simulink model "tadpole_dynamic_open_loop1"  (R2019b)
settings: Solver=ode4  StartTime=0.0  StopTime=sim_time  FixedStep=0.001  RelTol=1e-2
values from neighbouring files (symbols this model uses):
  C_alpha = 1000*ones(runcycle,1)    [rand_par.m]    (also in whole_par.m = 1000; whole_par_bias.m = 1000)
  C_beta = 50*ones(runcycle,1)    [rand_par.m]    (also in whole_par.m = 50; whole_par_bias.m = 50)
  Cd = 0.25*ones(runcycle,1)    [rand_par.m]    (also in whole_par.m = 0.25; whole_par_bias.m = 0.25)
  delta_fL = -1*ones(runcycle,1)    [rand_par.m]    (also in whole_par.m = -1; whole_par_bias.m = -1)
  delta_fR = 3.5*ones(runcycle,1)    [rand_par.m]    (also in whole_par.m = 3.5; whole_par_bias.m = 3.5)
  FA = 1*ones(runcycle,1)    [rand_par.m]    (also in whole_par.m = 1; whole_par_bias.m = 1)
  h = [ h(1:j-1) ; h(j+1:m)]    [UMDIRECT.m]    (also in whole_par.m = 0.4896; whole_par_bias.m = 0.4896)
  I_f_wheel = 0.3    [whole_par.m]    (also in whole_par_bias.m)
  I_r_wheel = 0.5    [whole_par.m]    (also in whole_par_bias.m)
  I_x = 12.1*ones(runcycle,1)    [rand_par.m]    (also in whole_par.m = 12.1; whole_par_bias.m = 12.1)
  I_y = 36.7*ones(runcycle,1)    [rand_par.m]    (also in whole_par.m = 36.7; whole_par_bias.m = 36.7)
  I_z = 50*DOE(:,2)    [rand_par.m]    (also in whole_par.m = 50; whole_par_bias.m = 60)
  k_z = 30000*ones(runcycle,1)    [rand_par.m]    (also in whole_par.m = 30000; whole_par_bias.m = 30000)
  l_1 = 0.724    [whole_par.m]    (also in whole_par_bias.m)
  l_2 = 0.719    [whole_par.m]    (also in whole_par_bias.m)
  m = m - 1    [UMDIRECT.m]    (also in rand_par.m = 48.3*DOE(:,1); whole_par.m = 48.3; whole_par_bias.m = 60)
  mu_dp = 0.8*ones(runcycle,1)    [rand_par.m]    (also in whole_par.m = 0.8; whole_par_bias.m = 0.8)
  mu_lp = 0.8*ones(runcycle,1)    [rand_par.m]    (also in whole_par.m = 0.8; whole_par_bias.m = 0.8)
  mu_rolling_1 = 0.009*ones(runcycle,1)    [rand_par.m]    (also in whole_par.m = 0.009; whole_par_bias.m = 0.009)
  mu_rolling_2 = 0.0005*ones(runcycle,1)    [rand_par.m]    (also in whole_par.m = 0.0005; whole_par_bias.m = 0.0005)
  R_0 = 0.335*ones(runcycle,1)    [rand_par.m]    (also in whole_par.m = 0.335; whole_par_bias.m = 0.335)
  rho = 1.225*ones(runcycle,1)    [rand_par.m]    (also in whole_par.m = 1.225; whole_par_bias.m = 1.225)
  SAP = 0.01*ones(runcycle,1)    [rand_par.m]    (also in whole_par.m = 0.01; whole_par_bias.m = 0.01)
  V_wind = 0*ones(runcycle,1)    [rand_par.m]    (also in whole_par.m = 0; whole_par_bias.m = 0)
libraries: simulink_extras x10, simulink x4
(part 1 of 4)
settings Model: Creator=yipin  LastModifiedBy=Chenyp
settings SolverCC: ZeroCrossAlgorithm=Adaptive  AlgebraicLoopSolver=LineSearch
settings DataIOCC: ReturnWorkspaceOutputs=off
settings DebuggingCC: MaxConsecutiveZCsMsg=warning  ArithmeticOperatorsInVariantConditions=warning
settings SFSimCC: CustomCodeUndefinedFunction=UseInterfaceOnly

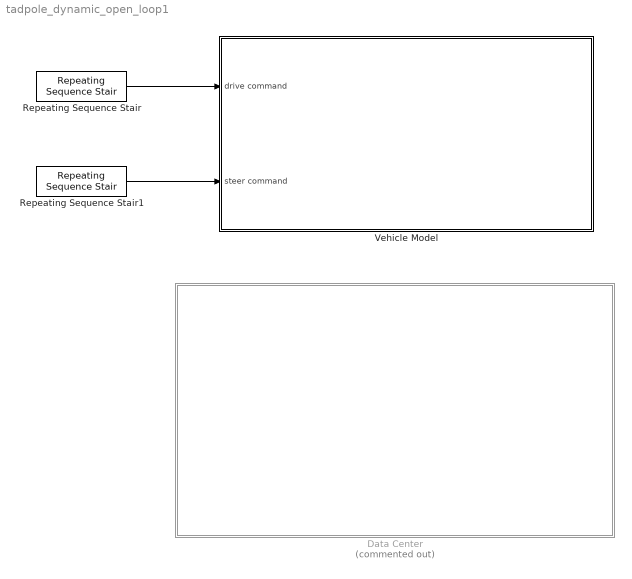
== system tadpole_dynamic_open_loop1 ==
  Data Center : Subsystem  Commented=on
  Repeating Sequence Stair : simulink/Sources/Repeating Sequence Stair  OutValues=drive_command  tsamp=-1  OutMin=[]  OutMax=[]  OutDataTypeStr=double  OutputDataTypeScalingMode=double  OutDataType=fixdt(0,8)  ConRadixGroup=Best Precision: Vector-wise  OutScaling=2^-12
  Repeating Sequence Stair1 : simulink/Sources/Repeating Sequence Stair  OutValues=steer_command  tsamp=-1  OutMin=[]  OutMax=[]  OutDataTypeStr=double  OutputDataTypeScalingMode=double  OutDataType=fixdt(0,8)  ConRadixGroup=Best Precision: Vector-wise  OutScaling=2^-12
  Vehicle Model : Subsystem
      mask Display: image('C:\Users\yipin\Desktop\擷取.PNG');
  wires:
  Repeating Sequence Stair/1 -> Vehicle Model/1("drive command ")
  Repeating Sequence Stair1/1 -> Vehicle Model/2(steer command)

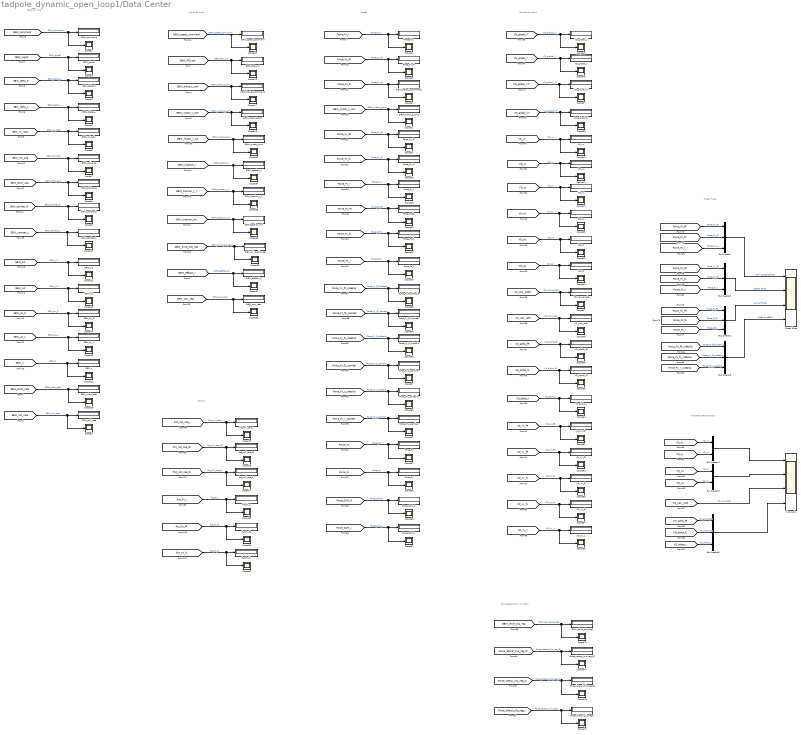
== system tadpole_dynamic_open_loop1/Data Center ==
  note: Steer By Wire
  note: Drive By Wire
  note: Vehicle Dynamic
  note: Forces
  note: Friction
  note: Wheel Force
  note: Kinematic Performance
  note: Slip Recgonition (-1 if slip)
  Bus Creator{,1..3,6} (5 alike) : BusCreator  Inputs=3
  Bus Creator4 : BusCreator  Inputs=2
  Bus Creator5 : BusCreator  Inputs=2
  DBW_PID_out : Display
  DBW_brake_t_command : Display
  DBW_brake_t_command1 : Display
  DBW_drive_slip_reg : Display
  DBW_drive_slip_reg1 : Display
  DBW_effRadi_R : Display
  DBW_motor_t_com : Display
  DBW_motor_t_com1 : Display
  DBW_motor_t_out : Display
  DBW_rpm_rear : Display
  DBW_speed_command : Display
  DBW_traction_out : Display
  DBW_traction_r : Display
  DBW_traction_r_T : Display
  Force_Fx : Display
  Force_Fx_fR : Display
  Force_Fx_r : Display
  Force_Fy : Display
  Force_Fy_fL : Display
  Force_Fy_fL_camber : Display
  Force_Fy_fL_sideslip : Display
  Force_Fy_fR : Display
  Force_Fy_fR_camber : Display
  Force_Fy_fR_sideslip : Display
  Force_Fy_r : Display
  Force_Fy_r_camber : Display
  Force_Fy_r_sideslip : Display
  Force_Fz_fL : Display
  Force_Fz_fR : Display
  Force_Fz_r : Display
  Force_SAM_L : Display
  Force_SAM_R : Display
  Force_lateral_slip_reg_fL : Display
  Force_lateral_slip_reg_fR : Display
  Force_lateral_slip_reg_r : Display
  SBW_an_L : Display
  SBW_an_R : Display
  SBW_camber_L : Display
  SBW_camber_R : Display
  SBW_command : Display
  SBW_delta_L : Display
  SBW_delta_R : Display
  SBW_h : Display
  SBW_pitch_ang : Display
  SBW_pitch_rate : Display
  SBW_roll_ang : Display
  SBW_roll_rate : Display
  SBW_signal : Display
  SBW_w1 : Display
  SBW_w2 : Display
  SBW_wl_ratio : Display
  Scope{1..64,66..68,73..82} (77 alike) : Scope
  VD_Ax : Display
  VD_Ay : Display
  VD_Az : Display
  VD_Vx_fL : Display
  VD_Vx_fR : Display
  VD_Vy_fL : Display
  VD_Vy_fR : Display
  VD_Vy_r : Display
  VD_alpha_fL : Display
  VD_alpha_fR : Display
  VD_alpha_r : Display
  VD_global_VX : Display
  VD_global_VY : Display
  VD_global_X : Display
  VD_global_Y : Display
  VD_vx : Display
  VD_vy : Display
  VD_vz : Display
  VD_yaw_angle : Display
  VD_yaw_rate : Display
  frct_Fx_fL : Display
  frct_Fx_fR : Display
  frct_Fx_r : Display
  frct_roll_coe_fL : Display
  frct_roll_coe_fR : Display
  frct_roll_coe_r : Display
  "kinematic " : Scope  NumInputPorts=4
  wheel force : Scope  NumInputPorts=4
  wires:
  [SBW_wl_ratio] -> Scope6/1, SBW_wl_ratio/1  "SBW_wl_ratio"
  [SBW_w2] -> Scope13/1, SBW_w2/1  "SBW_w2"
  [SBW_delta_L] -> Scope5/1, SBW_delta_L/1  "SBW_delta_L"
  [SBW_camber_R] -> Scope9/1, SBW_camber_R/1  "SBW_camber_R"
  [SBW_w1] -> Scope12/1, SBW_w1/1  "SBW_w1"
  [SBW_an_R] -> Scope14/1, SBW_an_R/1  "SBW_an_R"
  [SBW_signal] -> Scope3/1, SBW_signal/1  "SBW_signal"
  [SBW_pitch_ang] -> Scope8/1, SBW_pitch_ang/1  "SBW_pitch_ang"
  [SBW_an_L] -> Scope15/1, SBW_an_L/1  "SBW_an_L"
  [SBW_camber_L] -> Scope10/1, SBW_camber_L/1  "SBW_camber_L"
  [SBW_command] -> Scope1/1, SBW_command/1  "SBW_command"
  [SBW_delta_R] -> Scope4/1, SBW_delta_R/1  "SBW_dalta_R"
  [SBW_h] -> Scope11/1, SBW_h/1  "SBW_h"
  [SBW_roll_ang] -> Scope7/1, SBW_roll_ang/1  "SBW_roll_ang"
  [SBW_pitch_rate] -> Scope16/1, SBW_pitch_rate/1  "SBW_pitch_rate"
  [SBW_roll_rate] -> Scope2/1, SBW_roll_rate/1  "SBW_roll_rate"
  [DBW_PID_out] -> Scope19/1, DBW_PID_out/1  "DBW_PID_out"
  [DBW_motor_t_com] -> Scope18/1, DBW_motor_t_com/1  "DBW_motor_t_com"
  [DBW_brake_t_com] -> Scope17/1, DBW_brake_t_command/1  "DBW_brake_t_com"
  [DBW_speed_command] -> Scope20/1, DBW_speed_command/1  "DBW_speed_command"
  [Force_Fx_r] -> Scope24/1, Force_Fx_r/1  "Force_Fx_r"
  [DBW_motor_t_com] -> Scope22/1, DBW_motor_t_com1/1  "DBW_motor_t_com"
  [Force_Fx_fL] -> Scope21/1, DBW_brake_t_command1/1  "Force_Fx_fL"
  [Force_Fx_fR] -> Scope23/1, Force_Fx_fR/1  "Force_Fx_fR"
  [Force_Fy_fR] -> Scope27/1, Force_Fy_fR/1  "Force_Fy_fR"
  [Force_Fy_r] -> Scope26/1, Force_Fy_r/1  "Force_Fy_r"
  [Force_Fy_fL] -> Scope25/1, Force_Fy_fL/1  "Force_Fy_fL"
  [Force_Fz_r] -> Scope29/1, Force_Fz_r/1  "Force_Fz_r"
  [Force_Fz_fR] -> Scope30/1, Force_Fz_fR/1  "Force_Fz_fR"
  [Force_Fz_fL] -> Scope28/1, Force_Fz_fL/1  "Force_Fz_fL"
  [DBW_effRadi_r] -> Scope31/1, DBW_effRadi_R/1  "DBW_effRadi_R"
  [DPW_rpm_rear] -> Scope32/1, DBW_rpm_rear/1  "DBW_rpm_rear"
  [DBW_motor_t_out] -> Scope33/1, DBW_motor_t_out/1  "DBW_motor_t_out"
  [DBW_traction_r] -> Scope34/1, DBW_traction_r/1  "DBW_traction_r"
  [DBW_traction_r_T] -> Scope35/1, DBW_traction_r_T/1  "DBW_traction_r_T"
  [DBW_drive_slip_reg] -> Scope36/1, DBW_drive_slip_reg/1  "DBW_drive_slip_reg"
  [VD_Ay] -> Scope43/1, VD_Ay/1  "VD_Ay"
  [VD_Ax] -> Scope38/1, VD_Ax/1  "VD_Ax"
  [VD_global_VX] -> Scope37/1, VD_global_VX/1  "VD_global_VX"
  [VD_vz] -> Scope42/1, VD_vz/1  "VD_vz"
  [VD_global_VY] -> Scope39/1, VD_global_VY/1  "VD_global_VY"
  [VD_vy] -> Scope41/1, VD_vy/1  "VD_vy"
  [VD_vx] -> Scope40/1, VD_vx/1  "VD_vx"
  [VD_global_X] -> Scope45/1, VD_global_X/1  "VD_global_X"
  [VD_global_Y] -> Scope46/1, VD_global_Y/1  "VD_global_Y"
  [VD_Az] -> Scope44/1, VD_Az/1  "VD_Az"
  [VD_yaw_rate] -> Scope48/1, VD_yaw_rate/1  "VD_yaw_rate"
  [VD_yaw_angle] -> Scope47/1, VD_yaw_angle/1  "VD_yaw_angle"
  [VD_alpha_fR] -> Scope49/1, VD_alpha_fR/1  "VD_alpha_fR"
  [VD_alpha_fL] -> Scope50/1, VD_alpha_fL/1  "VD_alpha_fL"
  [VD_Vx_fL] -> Scope53/1, VD_Vx_fL/1  "VD_Vx_fL"
  [VD_Vy_fL] -> Scope54/1, VD_Vy_fL/1  "VD_Vy_fL"
  [VD_Vx_fR] -> Scope51/1, VD_Vx_fR/1  "VD_Vx_fR"
  [VD_Vy_fR] -> Scope52/1, VD_Vy_fR/1  "VD_Vy_fR"
  [Force_Fy_fR_sideslip] -> Scope55/1, Force_Fy_fR_sideslip/1  "Force_Fy_fR_sideslip"
  [Force_Fy_fR_camber] -> Scope58/1, Force_Fy_fR_camber/1  "Force_Fy_fR_camber"
  [Force_Fy_fL_sideslip] -> Scope56/1, Force_Fy_fL_sideslip/1  "Force_Fy_fL_sideslip"
  [Force_Fy_fL_camber] -> Scope57/1, Force_Fy_fL_camber/1  "Force_Fy_fL_camber"
  [VD_Vy_r] -> Scope59/1, VD_Vy_r/1  "VD_Vy_r"
  [Force_Fy_r_camber] -> Scope61/1, Force_Fy_r_camber/1  "Force_Fy_r_camber"
  [Force_Fy_r_sideslip] -> Scope60/1, Force_Fy_r_sideslip/1  "Force_Fy_r_sideslip"
  [Force_Fx] -> Scope62/1, Force_Fx/1  "Force_Fx"
  [Force_Fy] -> Scope63/1, Force_Fy/1  "Force_Fy"
  [Force_SAM_L] -> Scope67/1, Force_SAM_L/1  "Force_SAM_L"
  [Force_SAM_R] -> Scope66/1, Force_SAM_R/1  "Force_SAM_R"
  [DBW_traction_out] -> Scope68/1, DBW_traction_out/1  "DBW_traction_out"
  [Force_Fx_r_r] -> Bus Creator/3  "Force_Fx_r_r"
  [Force_Fx_fL] -> Bus Creator/2  "Force_Fx_fL"
  [Force_Fx_fR] -> Bus Creator/1  "Force_Fx_fR"
  [Force_Fy_fR] -> Bus Creator1/1  "Force_Fy_fR"
  [Force_Fy_fL] -> Bus Creator1/2  "Force_Fy_fL"
  [Force_Fz_fR] -> Bus Creator2/1  "Force_Fz_fR"
  [Force_Fz_fL] -> Bus Creator2/2  "Force_Fz_fL"
  [Force_Fz_r] -> Bus Creator2/3  "Force_Fz_r"
  [Force_Fy_fL_sideslip] -> Bus Creator3/2  "Force_Fy_fL_sideslip"
  [Force_Fy_fR_sideslip] -> Bus Creator3/1  "Force_Fy_fR_sideslip"
  [Force_Fy_r_sideslip] -> Bus Creator3/3  "Force_Fy_r_sideslip"
  Bus Creator/1 -> wheel force/1  "Rolling Resistance"
  Bus Creator1/1 -> wheel force/2  "Lateral Force"
  Bus Creator2/1 -> wheel force/3  "Normal Force"
  Bus Creator3/1 -> wheel force/4  "Sideslip effect"
  [Force_Fy_r] -> Bus Creator1/3  "Force_Fy_r"
  [VD_vy] -> Bus Creator4/2  "VD_vy"
  [VD_vx] -> Bus Creator4/1  "VD_vx"
  [VD_Ax] -> Bus Creator5/1  "VD_Ax"
  [VD_Ay] -> Bus Creator5/2  "VD_Ay"
  [VD_alpha_fR] -> Bus Creator6/1  "VD_alpha_fR"
  [VD_alpha_fL] -> Bus Creator6/2  "VD_alpha_fL"
  Bus Creator4/1 -> "kinematic "/1
  Bus Creator5/1 -> "kinematic "/2
  [VD_yaw_rate] -> "kinematic "/3  "VD_yaw_rate"
  Bus Creator6/1 -> "kinematic "/4
  [VD_alpha_r] -> Scope64/1, VD_alpha_r/1  "VD_alpha_r"
  [VD_alpha_r] -> Bus Creator6/3  "VD_alpha_r"
  [DBW_drive_slip_reg] -> Scope73/1, DBW_drive_slip_reg1/1  "DBW_drive_slip_reg"
  [Force_lateral_slip_reg_fR] -> Scope74/1, Force_lateral_slip_reg_fR/1  "Force_lateral_slip_reg_fR"
  [Force_lateral_slip_reg_fL] -> Scope75/1, Force_lateral_slip_reg_fL/1  "Force_lateral_slip_reg_fL"
  [Force_lateral_slip_reg_r] -> Scope76/1, Force_lateral_slip_reg_r/1  "Force_lateral_slip_reg_r"
  [frct_roll_coe_fL] -> Scope77/1, frct_roll_coe_fL/1  "frct_roll_coe_fL"
  [frct_roll_coe_fR] -> Scope78/1, frct_roll_coe_fR/1  "frct_roll_coe_fR"
  [frct_roll_coe_r] -> Scope79/1, frct_roll_coe_r/1  "frct_roll_coe_r"
  [frct_Fx_r] -> Scope80/1, frct_Fx_r/1  "frct_Fx_r"
  [frct_Fx_fR] -> Scope81/1, frct_Fx_fR/1  "frct_Fx_fR"
  [frct_Fx_fL] -> Scope82/1, frct_Fx_fL/1  "frct_Fx_fL"

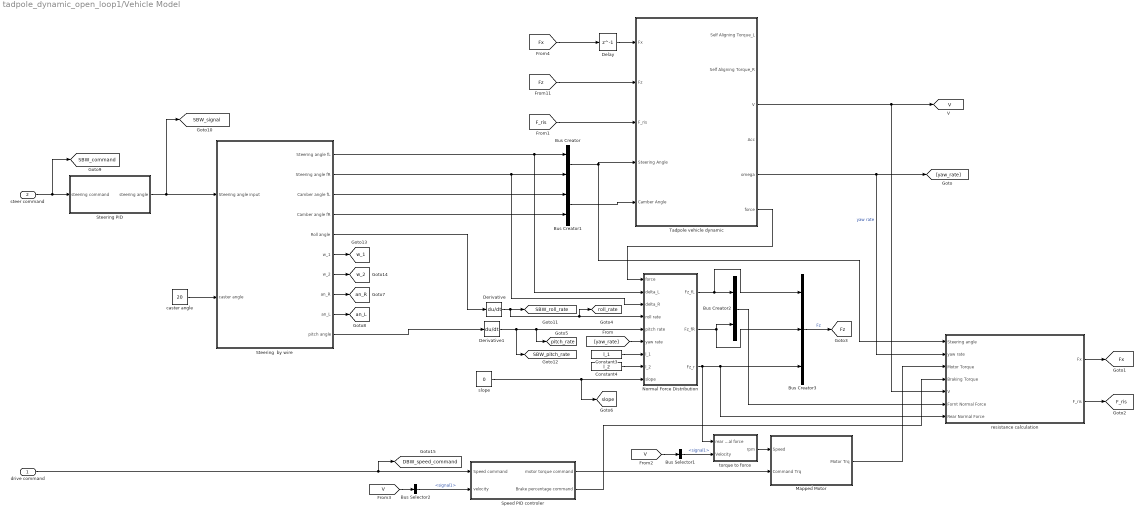
== system tadpole_dynamic_open_loop1/Vehicle Model ==
  "drive command " : Inport
  steer command : Inport  Port=2
  Bus Creator : BusCreator  Inputs=2
  Bus Creator1 : BusCreator  Inputs=2
  Bus Creator2 : BusCreator  Inputs=2
  Bus Creator3 : BusCreator  Inputs=3
  Bus Selector1 : BusSelector  OutputSignals=signal1
  Bus Selector2 : BusSelector  OutputSignals=signal1
  Constant3 : Constant  Value=l_1
  Constant4 : Constant  Value=l_2
  Delay : Delay  DelayLength=1  SampleTime=0.01
  Derivative : Derivative
  Derivative1 : Derivative
  Mapped Motor : Subsystem
  Normal Force Distribution : Subsystem
  "Speed PID controler " : Subsystem
  Steering  by wire : Subsystem  SystemSampleTime=469.048
  Steering PID : Subsystem
  Tadpole vehicle dynamic : Subsystem
  caster angle : Constant  Value=20
  resistance calculation : Subsystem
  slope : Constant  Value=0
  torque to force : Subsystem
  tag scope: DBW_speed_command=global, F_ris=global, Fx=global, Fz=global, SBW_command=global, SBW_pitch_rate=global, SBW_roll_rate=global, SBW_signal=global, V=global, an_L=global, an_R=global, pitch_rate=global, roll_rate=global, slope=global, w_1=global, w_2=global
  wires:
  Steering PID/1("steering angle ") -> [SBW_signal], Steering  by wire/1(Steering angle input)
  Bus Creator/1 -> Tadpole vehicle dynamic/4(Steering Angle), resistance calculation/1(Steering angle)
  Steering  by wire/2(Steering angle fR) -> Normal Force Distribution/3(delta_R), Bus Creator/2
  Steering  by wire/1(Steering angle fL) -> Normal Force Distribution/2(delta_L), Bus Creator/1
  steer command/1 -> [SBW_command], Steering PID/1(steering command)
  caster angle/1 -> Steering  by wire/2(caster angle)
  Steering  by wire/3(Camber angle fL) -> Bus Creator1/1
  Steering  by wire/4(Camber angle fR) -> Bus Creator1/2
  Bus Creator1/1 -> Tadpole vehicle dynamic/5(Camber Angle)
  Tadpole vehicle dynamic/5(omega) -> resistance calculation/2(yaw rate), [yaw_rate]  "yaw rate"
  Steering  by wire/6(w_1) -> [w_1]
  Steering  by wire/7(w_2) -> [w_2]
  [Fz] -> Tadpole vehicle dynamic/2(Fz)
  Derivative/1 -> [SBW_roll_rate], Normal Force Distribution/4(roll rate), [roll_rate]
  Derivative1/1 -> [SBW_pitch_rate], Normal Force Distribution/5(pitch rate), [pitch_rate]
  [yaw_rate] -> Normal Force Distribution/6(yaw rate)
  Steering  by wire/5(Roll angle) -> Derivative/1
  Steering  by wire/10(pitch angle) -> Derivative1/1
  Constant3/1 -> Normal Force Distribution/7(l_1)
  Constant4/1 -> Normal Force Distribution/8(l_2)
  Normal Force Distribution/1(Fz_fL) -> Bus Creator3/1, Bus Creator2/1
  Normal Force Distribution/2(Fz_fR) -> Bus Creator2/2, Bus Creator3/2
  Bus Creator2/1 -> resistance calculation/6("Fornt Normal Force ")
  Normal Force Distribution/3(Fz_r) -> Bus Creator3/3, resistance calculation/7(Rear Normal Force), torque to force/1(rear normal force)
  Bus Creator3/1 -> [Fz]  "Fz"
  slope/1 -> Normal Force Distribution/9(slope), [slope]
  resistance calculation/2(F_ris) -> [F_ris]
  [F_ris] -> Tadpole vehicle dynamic/3(F_ris)
  Mapped Motor/1(Motor Trq) -> resistance calculation/3("Motor Torque ")
  [V] -> Bus Selector1/1
  Bus Selector1/1 -> torque to force/2(Velocity)  "<signal1>"
  torque to force/1(rpm) -> Mapped Motor/1(Speed)
  [V] -> Bus Selector2/1
  Bus Selector2/1 -> "Speed PID controler "/2(velocity)  "<signal1>"
  "Speed PID controler "/1("motor torque command ") -> Mapped Motor/2(Command Trq)
  "drive command "/1 -> [DBW_speed_command], "Speed PID controler "/1(Speed command)
  Tadpole vehicle dynamic/6(force) -> Normal Force Distribution/1(force)
  "Speed PID controler "/2(Brake percentage command) -> resistance calculation/4("Braking Torque ")
  [Fx] -> Delay/1
  resistance calculation/1(Fx) -> [Fx]
  Delay/1 -> Tadpole vehicle dynamic/1(Fx)
  Steering  by wire/8(an_R) -> [an_R]
  Steering  by wire/9(an_L) -> [an_L]
  Tadpole vehicle dynamic/3(V) -> resistance calculation/5(V), [V]

== system tadpole_dynamic_open_loop1/Vehicle Model/Mapped Motor ==
  note: response time
  note: 將一段時間(Tc)的頻率做積分，其中的gain值為Tc的倒數
  note: 查表得知在給定轉速的扭力上限，其中Table Data(N*m)為扭力上限值，而Breakpoints(rad/s)為對應的轉速。
  note: 大於一就為一，小於負一就為負一。
  Speed : Inport
  Command Trq : Inport  Port=2
  1-D Lookup Table1 : Lookup_n-D  NumberOfTableDimensions=1  BreakpointsForDimension1=[299,300,303,307,308,310,311,314,316,319,322,324,327,331,335,338,339,341,346,348,350,355,360,365,370,371,372,376,377,380,383,384,386,388,389,390]  Table=[20.43,19.9,19.46,18.88,18.23,17.61,16.9,16.21,15.55,14.87,14.19,13.51,12.83,12.16,11.46,10.83,10.12,9.45,8.82,8.19,7.56,6.96,5.82,4.75,3.82,3.39,2.94,2.54,2.24,1.63,1.33,0.75,0.59,0.45,0.08,0.04]  InternalRulePriority=Speed  RndMeth=Simplest  InputSameDT=on
  Divide2 : Product
  Gain1 : Gain  Gain=100
  Integrator : Integrator
  Interpolated zero-crossing : Lookup_n-D  NumberOfTableDimensions=1  BreakpointsForDimension1=[-1 1]  Table=[-1 1]  ExtrapMethod=Clip  InternalRulePriority=Speed  RndMeth=Simplest  InputSameDT=on
  Product : Product  Inputs=/*
  Sum : Sum  Inputs=|+-
  Motor Trq : Outport  VectorParamsAs1DForOutWhenUnconnected=off
  tag scope: DBW_motor_t_out=global
  wires:
  Product/1 -> Interpolated zero-crossing/1
  Gain1/1 -> Product/2, Sum/2
  Sum/1 -> Integrator/1
  Divide2/1 -> [DBW_motor_t_out], Motor Trq/1  "integral"
  Integrator/1 -> Gain1/1
  1-D Lookup Table1/1 -> Product/1, Divide2/1
  Interpolated zero-crossing/1 -> Divide2/2
  Command Trq/1 -> Sum/1  "cmd"
  Speed/1 -> 1-D Lookup Table1/1

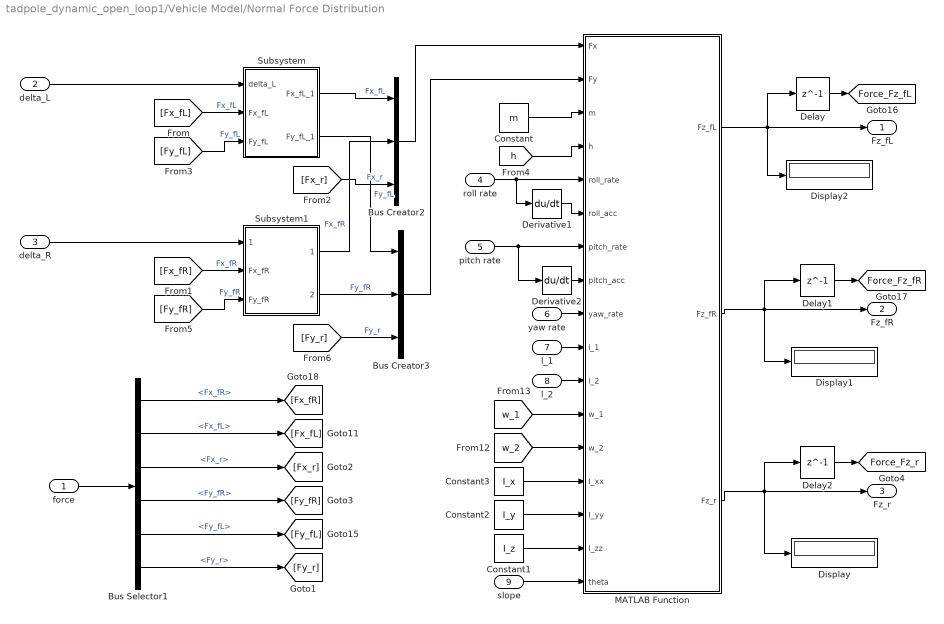
== system tadpole_dynamic_open_loop1/Vehicle Model/Normal Force Distribution ==
  force : Inport
  delta_L : Inport  Port=2
  delta_R : Inport  Port=3
  roll rate : Inport  Port=4
  pitch rate : Inport  Port=5
  yaw rate : Inport  Port=6
  l_1 : Inport  Port=7
  l_2 : Inport  Port=8
  slope : Inport  Port=9
  Bus Creator2 : BusCreator  Inputs=3
  Bus Creator3 : BusCreator  Inputs=3
  Bus Selector1 : BusSelector  OutputSignals=Fx_fR,Fx_fL,Fx_r,Fy_fR,Fy_fL,Fy_r
  Constant : Constant  Value=m
  Constant1 : Constant  Value=I_z
  Constant2 : Constant  Value=I_y
  Constant3 : Constant  Value=I_x
  Delay : Delay  DelayLength=1
  Delay1 : Delay  DelayLength=1
  Delay2 : Delay  DelayLength=1
  Derivative1 : Derivative
  Derivative2 : Derivative
  Display : Display
  Display1 : Display
  Display2 : Display
  MATLAB Function : MATLAB Function  TreatAsAtomicUnit=on
  Subsystem : Subsystem
  Subsystem1 : Subsystem
  Fz_fL : Outport  VectorParamsAs1DForOutWhenUnconnected=off
  Fz_fR : Outport  Port=2  VectorParamsAs1DForOutWhenUnconnected=off
  Fz_r : Outport  Port=3  VectorParamsAs1DForOutWhenUnconnected=off
  tag scope: Force_Fz_fL=global, Force_Fz_fR=global, Force_Fz_r=global
  wires:
  pitch rate/1 -> Derivative2/1, MATLAB Function/7(pitch_rate)
  yaw rate/1 -> MATLAB Function/9(yaw_rate)
  Bus Creator2/1 -> MATLAB Function/1(Fx)
  [Fx_fL] -> Subsystem/2(Fx_fL)  "Fx_fL"
  [Fx_r] -> Bus Creator2/3  "Fx_r"
  Constant3/1 -> MATLAB Function/14(I_xx)
  [w_1] -> MATLAB Function/12(w_1)
  Constant1/1 -> MATLAB Function/16(I_zz)
  delta_R/1 -> Subsystem1/1(delta_R)
  Subsystem/1(Fx_fL_1) -> Bus Creator2/1  "Fx_fL"
  Subsystem1/2(Fy_fR_1) -> Bus Creator3/2  "Fy_fR"
  roll rate/1 -> Derivative1/1, MATLAB Function/5(roll_rate)
  Constant/1 -> MATLAB Function/3(m)
  Bus Creator3/1 -> MATLAB Function/2(Fy)
  [Fy_fL] -> Subsystem/3(Fy_fL)  "Fy_fL"
  Constant2/1 -> MATLAB Function/15(I_yy)
  [Fx_fR] -> Subsystem1/2(Fx_fR)  "Fx_fR"
  [w_2] -> MATLAB Function/13(w_2)
  Subsystem/2(Fy_fL_1) -> Bus Creator3/1  "Fy_fL"
  l_1/1 -> MATLAB Function/10(l_1)
  [Fy_r] -> Bus Creator3/3  "Fy_r"
  l_2/1 -> MATLAB Function/11(l_2)
  [Fy_fR] -> Subsystem1/3(Fy_fR)  "Fy_fR"
  Subsystem1/1(Fx_fR_1) -> Bus Creator2/2  "Fx_fR"
  [h] -> MATLAB Function/4(h)
  delta_L/1 -> Subsystem/1(delta_L)
  slope/1 -> MATLAB Function/17(theta)
  Bus Selector1/5 -> [Fy_fL]  "<Fy_fL>"
  Bus Selector1/4 -> [Fy_fR]  "<Fy_fR>"
  Bus Selector1/6 -> [Fy_r]  "<Fy_r>"
  Bus Selector1/2 -> [Fx_fL]  "<Fx_fL>"
  Bus Selector1/1 -> [Fx_fR]  "<Fx_fR>"
  Bus Selector1/3 -> [Fx_r]  "<Fx_r>"
  force/1 -> Bus Selector1/1
  MATLAB Function/2(Fz_fR) -> Fz_fR/1, Delay1/1, Display1/1
  MATLAB Function/3(Fz_r) -> Delay2/1, Display/1, Fz_r/1
  MATLAB Function/1(Fz_fL) -> Delay/1, Display2/1, Fz_fL/1
  Delay/1 -> [Force_Fz_fL]
  Delay1/1 -> [Force_Fz_fR]
  Delay2/1 -> [Force_Fz_r]
  Derivative1/1 -> MATLAB Function/6(roll_acc)
  Derivative2/1 -> MATLAB Function/8(pitch_acc)

== system tadpole_dynamic_open_loop1/Vehicle Model/Speed PID controler  ==
  Speed command : Inport
  velocity : Inport  Port=2
  Gain : Gain  Gain=-1
  Gain1 : Gain
  If : If
  If Action Subsystem : Subsystem  TreatAsAtomicUnit=on
  If Action Subsystem1 : Subsystem  TreatAsAtomicUnit=on
  PID : Subsystem
  Saturation1 : Saturate  UpperLimit=20  LowerLimit=0-0.5
  Saturation2 : Saturate  UpperLimit=0  LowerLimit=-10
  Sum1 : Sum  Inputs=|+-
  "motor torque command " : Outport  VectorParamsAs1DForOutWhenUnconnected=off
  Brake percentage command : Outport  Port=2  VectorParamsAs1DForOutWhenUnconnected=off
  tag scope: DBW_PID_out=global, DBW_brake_t_com=global, DBW_motor_t_com=global
  wires:
  Gain1/1 -> PID/1(R(s))
  Speed command/1 -> Sum1/1
  Sum1/1 -> Gain1/1
  velocity/1 -> Sum1/2
  PID/1(C(s)) -> [DBW_PID_out], If/1, If Action Subsystem1/1(In1), If Action Subsystem/1(In1)
  If/1 -> If Action Subsystem/Action
  If Action Subsystem/1(Out1) -> Saturation1/1
  Saturation1/1 -> [DBW_motor_t_com], "motor torque command "/1
  If/2 -> If Action Subsystem1/Action
  If Action Subsystem1/1(Out1) -> Saturation2/1
  Saturation2/1 -> Gain/1
  Gain/1 -> [DBW_brake_t_com], Brake percentage command/1

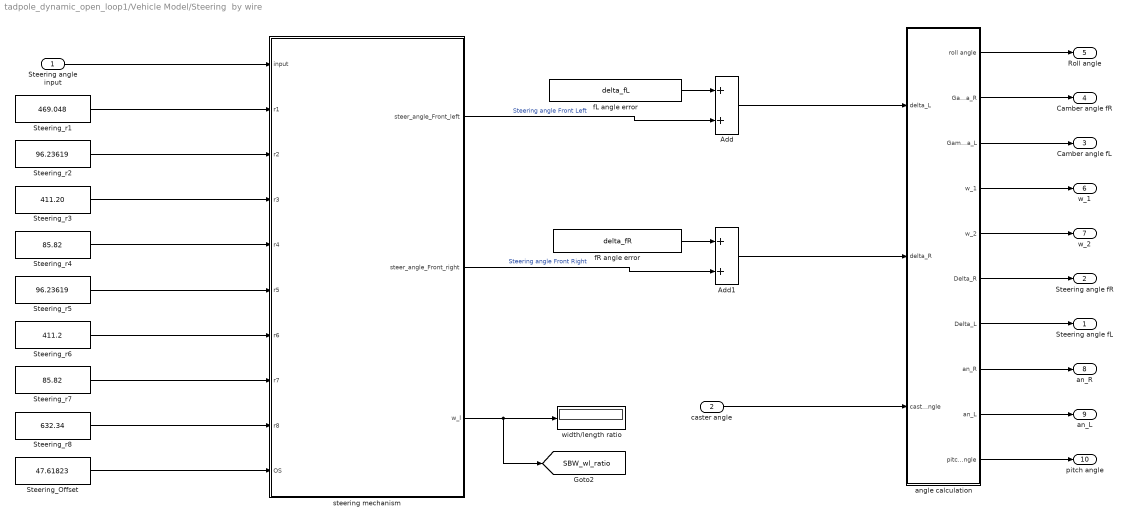
== system tadpole_dynamic_open_loop1/Vehicle Model/Steering  by wire ==
  Steering angle input : Inport
  caster angle : Inport  Port=2
  Add : Sum
  Add1 : Sum
  Steering_Offset : Constant  Value=47.61823
  Steering_r1 : Constant  Value=469.048
  Steering_r2 : Constant  Value=96.23619
  Steering_r3 : Constant  Value=411.20
  Steering_r4 : Constant  Value=85.82
  Steering_r5 : Constant  Value=96.23619
  Steering_r6 : Constant  Value=411.2
  Steering_r7 : Constant  Value=85.82
  Steering_r8 : Constant  Value=632.34
  angle calculation : Subsystem
  fL angle error : Constant  Value=delta_fL
  fR angle error : Constant  Value=delta_fR
  steering mechanism : MATLAB Function  TreatAsAtomicUnit=on
  width/length ratio : Display
  Steering angle fL : Outport  VectorParamsAs1DForOutWhenUnconnected=off
  Steering angle fR : Outport  Port=2  VectorParamsAs1DForOutWhenUnconnected=off
  Camber angle fL : Outport  Port=3  VectorParamsAs1DForOutWhenUnconnected=off
  Camber angle fR : Outport  Port=4  VectorParamsAs1DForOutWhenUnconnected=off
  Roll angle : Outport  Port=5  VectorParamsAs1DForOutWhenUnconnected=off
  w_1 : Outport  Port=6  VectorParamsAs1DForOutWhenUnconnected=off
  w_2 : Outport  Port=7  VectorParamsAs1DForOutWhenUnconnected=off
  an_R : Outport  Port=8  VectorParamsAs1DForOutWhenUnconnected=off
  an_L : Outport  Port=9  VectorParamsAs1DForOutWhenUnconnected=off
  pitch angle : Outport  Port=10  VectorParamsAs1DForOutWhenUnconnected=off
  tag scope: SBW_wl_ratio=global
  wires:
  Steering_r7/1 -> steering mechanism/8(r7)
  Steering_r5/1 -> steering mechanism/6(r5)
  Steering_Offset/1 -> steering mechanism/10(OS)
  Steering_r1/1 -> steering mechanism/2(r1)
  Steering_r4/1 -> steering mechanism/5(r4)
  Steering_r6/1 -> steering mechanism/7(r6)
  Steering_r3/1 -> steering mechanism/4(r3)
  Steering_r2/1 -> steering mechanism/3(r2)
  Steering_r8/1 -> steering mechanism/9(r8)
  Steering angle input/1 -> steering mechanism/1(input)
  steering mechanism/1(steer_angle_Front_left) -> Add/2  "Steering angle Front Left"
  steering mechanism/2(steer_angle_Front_right) -> Add1/2  "Steering angle Front Right"
  steering mechanism/3(w_l) -> [SBW_wl_ratio], width/length ratio/1
  fL angle error/1 -> Add/1
  fR angle error/1 -> Add1/1
  Add/1 -> angle calculation/1(delta_L)
  Add1/1 -> angle calculation/2(delta_R)
  caster angle/1 -> angle calculation/3(caster angle)
  angle calculation/7(Delta_L) -> Steering angle fL/1
  angle calculation/6(Delta_R) -> Steering angle fR/1
  angle calculation/2(Gamma_R) -> Camber angle fR/1
  angle calculation/3(Gamma_L) -> Camber angle fL/1
  angle calculation/1(roll angle) -> Roll angle/1
  angle calculation/4(w_1) -> w_1/1
  angle calculation/5(w_2) -> w_2/1
  angle calculation/8(an_R) -> an_R/1
  angle calculation/9(an_L) -> an_L/1
  angle calculation/10(pitch angle) -> pitch angle/1

== system tadpole_dynamic_open_loop1/Vehicle Model/Steering PID ==
  steering command : Inport
  Sum : Sum  Inputs=|+-
  steering angle PID : simulink/Continuous/PID Controller  Controller=PID  Form=Parallel  TimeDomain=Continuous-time  SampleTime=-1  IntegratorMethod=Forward Euler  FilterMethod=Forward Euler  ControllerParametersSource=internal  P=0  I=8  D=0  UseFilter=on  N=100  TunerSelectOption=Transfer Function Based (PID Tuner App)  InitialConditionSource=internal  InitialConditionForIntegrator=0  InitialConditionForFilter=0  DifferentiatorICPrevScaledInput=0  ExternalReset=none  TrackingMode=off  Kt=1  LimitOutput=off  UpperSaturationLimit=inf  LowerSaturationLimit=-inf  LinearizeAsGain=on  AntiWindupMode=none  Kb=1  POutMin=[]  POutMax=[]  IOutMin=[]  IOutMax=[]  DOutMin=[]  DOutMax=[]  NOutMin=[]  NOutMax=[]  SumOutMin=[]  SumOutMax=[]  SaturationOutMin=[]  SaturationOutMax=[]  PParamMin=[]  PParamMax=[]  IParamMin=[]  IParamMax=[]  DParamMin=[]  DParamMax=[]  NParamMin=[]  NParamMax=[]  KbParamMin=[]  KbParamMax=[]  KtParamMin=[]  KtParamMax=[]  KbOutMin=[]  KbOutMax=[]  KtOutMin=[]  KtOutMax=[]  IntegratorOutMin=[]  IntegratorOutMax=[]  FilterOutMin=[]  FilterOutMax=[]  SumI1OutMin=[]  SumI1OutMax=[]  SumI2OutMin=[]  SumI2OutMax=[]  SumI3OutMin=[]  SumI3OutMax=[]  SumI4OutMin=[]  SumI4OutMax=[]  SumDOutMin=[]  SumDOutMax=[]  DifferentiatorOutMin=[]  DifferentiatorOutMax=[]  FilterDiffOutCoefMin=[]  FilterDiffOutCoefMax=[]  ReciprocalOutMin=[]  ReciprocalOutMax=[]  SumDenOutMin=[]  SumDenOutMax=[]  SumNumOutMin=[]  SumNumOutMax=[]  DivideOutMin=[]  DivideOutMax=[]  IntegratorContinuousStateAttributes=''  IntegratorStateMustResolveToSignalObject=off  IntegratorRTWStateStorageClass=Auto  FilterContinuousStateAttributes=''  FilterStateMustResolveToSignalObject=off  FilterRTWStateStorageClass=Auto  ParallelPVariant=InternalParameters  IdealPVariant=Disabled  IVariant=InternalParameters  DVariant=InternalParameters  IntegratorVariant=Continuous  SatVariant=Disabled  AWVariant=Passthrough  PCopyVariant=Disabled  TRVariant=Disabled  FdbkBlocksVariant=Forward  IdealPFdbkVariant=Disabled  SatFdbkVariant=Disabled  DerivativeFilterVariant=ContFilter  NVariant=InternalParameters  NCopyVariant=Disabled  FilterICVariant=InternalICsFilter  IntegratorICVariant=InternalICs  ExternalResetVariant=Disabled  TRSumVariant=Passthrough  SumFdbkVariant=Disabled  SumVariant=Sum_PID
  steering command limit : Saturate  UpperLimit=50  LowerLimit=-50
  "steering angle " : Outport  VectorParamsAs1DForOutWhenUnconnected=off
  wires:
  steering command/1 -> steering command limit/1
  steering angle PID/1 -> Sum/2, "steering angle "/1
  steering command limit/1 -> Sum/1
  Sum/1 -> steering angle PID/1

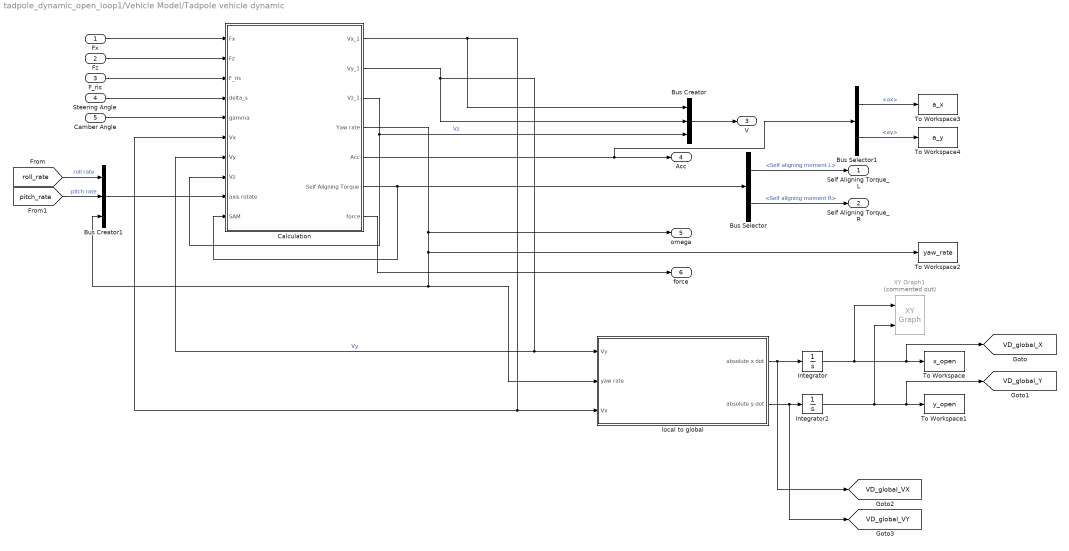
== system tadpole_dynamic_open_loop1/Vehicle Model/Tadpole vehicle dynamic ==
  Fx : Inport
  Fz : Inport  Port=2
  F_ris : Inport  Port=3
  Steering Angle : Inport  Port=4
  Camber Angle : Inport  Port=5
  Bus Creator : BusCreator  Inputs=3
  Bus Creator1 : BusCreator  Inputs=3
  Bus Selector : BusSelector  OutputSignals=Self aligning moment L,Self aligning moment R
  Bus Selector1 : BusSelector  OutputSignals=ax,ay
  Calculation : Subsystem
  Integrator : Integrator
  Integrator2 : Integrator
  To Workspace : ToWorkspace  VariableName=x_open  SaveFormat=Timeseries  SampleTime=-1
  To Workspace1 : ToWorkspace  VariableName=y_open  SaveFormat=Timeseries  SampleTime=-1
  To Workspace2 : ToWorkspace  VariableName=yaw_rate  SaveFormat=Timeseries  SampleTime=-1
  To Workspace3 : ToWorkspace  VariableName=a_x  SaveFormat=Timeseries  SampleTime=-1
  To Workspace4 : ToWorkspace  VariableName=a_y  SaveFormat=Timeseries  SampleTime=-1
  XY Graph1 : simulink/Sinks/XY Graph  Commented=on  xmin=-10  xmax=40  ymin=-30  ymax=30  st=-1
  local to global : Subsystem
  Self Aligning Torque_L : Outport  VectorParamsAs1DForOutWhenUnconnected=off
  Self Aligning Torque_R : Outport  Port=2  VectorParamsAs1DForOutWhenUnconnected=off
  V : Outport  Port=3  VectorParamsAs1DForOutWhenUnconnected=off
  Acc : Outport  Port=4  VectorParamsAs1DForOutWhenUnconnected=off
  omega : Outport  Port=5  VectorParamsAs1DForOutWhenUnconnected=off
  force : Outport  Port=6  VectorParamsAs1DForOutWhenUnconnected=off
  tag scope: VD_global_VX=global, VD_global_VY=global, VD_global_X=global, VD_global_Y=global
  wires:
  local to global/1(absolute x dot) -> [VD_global_VX], Integrator/1
  Integrator2/1 -> [VD_global_Y], To Workspace1/1, XY Graph1/2
  local to global/2(absolute y dot) -> [VD_global_VY], Integrator2/1
  Integrator/1 -> XY Graph1/1, [VD_global_X], To Workspace/1
  Calculation/1(Vx_1) -> Bus Creator/1, Calculation/6(Vx), local to global/3(Vx)
  Calculation/2(Vy_1) -> Bus Creator/2, Calculation/7(Vy), local to global/1(Vy)  "Vy"
  Calculation/4(Yaw rate) -> omega/1, Bus Creator1/3, local to global/2(yaw rate), To Workspace2/1
  Calculation/5(Acc) -> Bus Selector1/1, Acc/1
  Fx/1 -> Calculation/1(Fx)
  Steering Angle/1 -> Calculation/4(delta_s)
  Calculation/6(Self Aligning Torque) -> Calculation/10(SAM), Bus Selector/1
  Fz/1 -> Calculation/2(Fz)
  Bus Selector/2 -> Self Aligning Torque_R/1  "<Self aligning moment R>"
  Bus Selector/1 -> Self Aligning Torque_L/1  "<Self aligning moment L>"
  Camber Angle/1 -> Calculation/5(gamma)
  Calculation/3(Vz_1) -> Calculation/8(Vz), Bus Creator/3  "Vz"
  Bus Creator/1 -> V/1
  F_ris/1 -> Calculation/3(F_ris)
  [roll_rate] -> Bus Creator1/1  "roll rate"
  [pitch_rate] -> Bus Creator1/2  "pitch rate"
  Bus Creator1/1 -> Calculation/9(axis rotate)
  Calculation/7(force) -> force/1
  Bus Selector1/1 -> To Workspace3/1  "<ax>"
  Bus Selector1/2 -> To Workspace4/1  "<ay>"

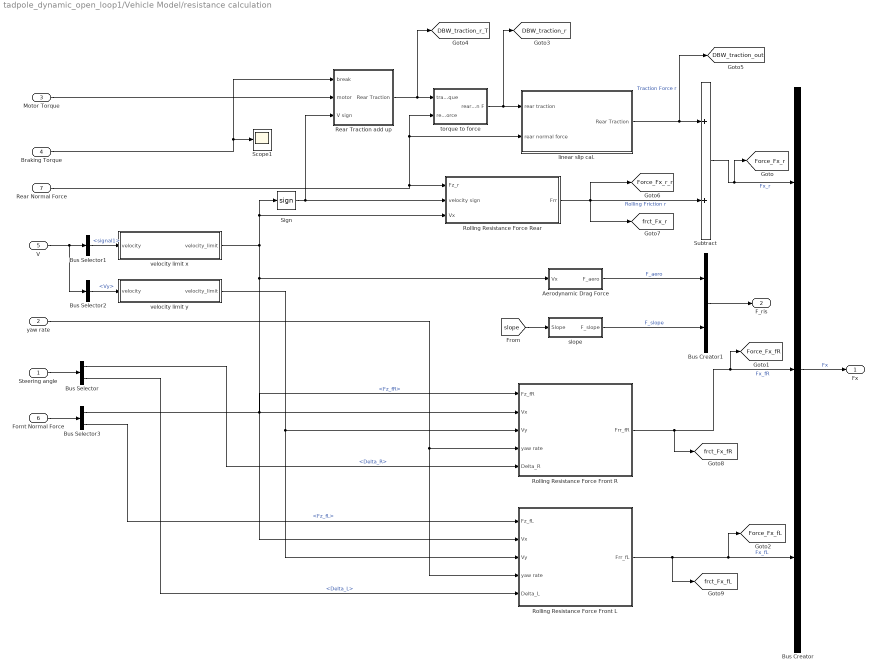
== system tadpole_dynamic_open_loop1/Vehicle Model/resistance calculation ==
  Steering angle : Inport
  yaw rate : Inport  Port=2
  "Motor Torque " : Inport  Port=3
  "Braking Torque " : Inport  Port=4
  V : Inport  Port=5
  "Fornt Normal Force " : Inport  Port=6
  Rear Normal Force : Inport  Port=7
  Aerodynamic Drag Force : Subsystem
  Bus Creator : BusCreator  Inputs=3
  Bus Creator1 : BusCreator  Inputs=2
  Bus Selector : BusSelector  OutputSignals=Delta_R,Delta_L
  Bus Selector1 : BusSelector  OutputSignals=signal1
  Bus Selector2 : BusSelector  OutputSignals=Vy
  Bus Selector3 : BusSelector  OutputSignals=Fz_fR,Fz_fL
  Rear Traction add up : Subsystem
  Rolling Resistance Force Front L : Subsystem
  Rolling Resistance Force Front R : Subsystem
  Rolling Resistance Force Rear : Subsystem
  Scope1 : Scope
  Sign : Signum
  Subtract : Sum
  "linear slip cal. " : Subsystem
  "slope " : Subsystem
  torque to force : Subsystem
  velocity limit x : Subsystem
  velocity limit y : Subsystem
  Fx : Outport  VectorParamsAs1DForOutWhenUnconnected=off
  F_ris : Outport  Port=2  VectorParamsAs1DForOutWhenUnconnected=off
  tag scope: DBW_traction_out=global, DBW_traction_r=global, DBW_traction_r_T=global, Force_Fx_fL=global, Force_Fx_fR=global, Force_Fx_r=global, Force_Fx_r_r=global, frct_Fx_fL=global, frct_Fx_fR=global, frct_Fx_r=global
  wires:
  Subtract/1 -> [Force_Fx_r], Bus Creator/1  "Fx_r"
  Sign/1 -> Rear Traction add up/3(V sign), Rolling Resistance Force Rear/2(velocity sign)
  "Braking Torque "/1 -> Rear Traction add up/1(break), Scope1/1
  Rear Traction add up/1(Rear Traction) -> [DBW_traction_r_T], torque to force/1(traction torque)
  "linear slip cal. "/1("Rear Traction ") -> [DBW_traction_out], Subtract/1  "Traction Force r"
  "Fornt Normal Force "/1 -> Bus Selector3/1
  Rear Normal Force/1 -> torque to force/2(rear normal force), "linear slip cal. "/2(rear normal force), Rolling Resistance Force Rear/1(Fz_r)
  V/1 -> Bus Selector2/1, Bus Selector1/1
  velocity limit x/1("velocity_limit ") -> Sign/1, Rolling Resistance Force Rear/3(Vx), Aerodynamic Drag Force/1(Vx), Rolling Resistance Force Front L/2(Vx), Rolling Resistance Force Front R/2(Vx)
  Rolling Resistance Force Rear/1(Frr) -> [frct_Fx_r], [Force_Fx_r_r], Subtract/2  "Rolling Friction r"
  [slope] -> "slope "/1(Slope)
  "Motor Torque "/1 -> Rear Traction add up/2(motor)
  torque to force/1(rear traction F) -> [DBW_traction_r], "linear slip cal. "/1(rear traction)
  Bus Selector1/1 -> velocity limit x/1("velocity ")  "<signal1>"
  Bus Selector2/1 -> velocity limit y/1("velocity ")  "<Vy>"
  Steering angle/1 -> Bus Selector/1
  Bus Selector/1 -> Rolling Resistance Force Front R/5(Delta_R)  "<Delta_R>"
  velocity limit y/1("velocity_limit ") -> Rolling Resistance Force Front L/3(Vy), Rolling Resistance Force Front R/3(Vy)
  yaw rate/1 -> Rolling Resistance Force Front L/4(yaw rate), Rolling Resistance Force Front R/4(yaw rate)
  Bus Selector/2 -> Rolling Resistance Force Front L/5(Delta_L)  "<Delta_L>"
  Bus Selector3/1 -> Rolling Resistance Force Front R/1(Fz_fR)  "<Fz_fR>"
  Bus Selector3/2 -> Rolling Resistance Force Front L/1(Fz_fL)  "<Fz_fL>"
  "slope "/1(F_slope) -> Bus Creator1/2  "F_slope"
  Rolling Resistance Force Front R/1(Frr_fR) -> [frct_Fx_fR], [Force_Fx_fR], Bus Creator/2  "Fx_fR"
  Rolling Resistance Force Front L/1(Frr_fL) -> [frct_Fx_fL], [Force_Fx_fL], Bus Creator/3  "Fx_fL"
  Bus Creator/1 -> Fx/1  "Fx"
  Aerodynamic Drag Force/1(F_aero) -> Bus Creator1/1  "F_aero"
  Bus Creator1/1 -> F_ris/1

== system tadpole_dynamic_open_loop1/Vehicle Model/torque to force ==
  rear normal force : Inport
  Velocity : Inport  Port=2
  Add : Sum  Inputs=+-
  Divide1 : Product  Inputs=*/
  Divide2 : Product  Inputs=*/
  Initial wheel radius : Constant  Value=R_0
  rad/s to rpm : Gain  Gain=60/2/pi
  tire vertical stiffness : Constant  Value=k_z
  rpm : Outport  VectorParamsAs1DForOutWhenUnconnected=off
  tag scope: DBW_effRadi_r=global, DPW_rpm_rear=global
  wires:
  Velocity/1 -> Divide1/1
  Divide1/1 -> rad/s to rpm/1
  tire vertical stiffness/1 -> Divide2/2
  rear normal force/1 -> Divide2/1
  Divide2/1 -> Add/2
  Initial wheel radius/1 -> Add/1
  Add/1 -> [DBW_effRadi_r], Divide1/2  "effective radius"
  rad/s to rpm/1 -> [DPW_rpm_rear], rpm/1

== system tadpole_dynamic_open_loop1/Vehicle Model/Normal Force Distribution/Subsystem ==
  delta_L : Inport
  Fx_fL : Inport  Port=2
  Fy_fL : Inport  Port=3
  Add : Sum  Inputs=+-
  Add1 : Sum
  Cos : Trigonometry  Operator=cos
  Product{,1..3} (4 alike) : Product
  Sin : Trigonometry
  Fx_fL_1 : Outport  VectorParamsAs1DForOutWhenUnconnected=off
  Fy_fL_1 : Outport  Port=2  VectorParamsAs1DForOutWhenUnconnected=off
  wires:
  delta_L/1 -> Sin/1, Cos/1
  Fx_fL/1 -> Product/2, Product2/2
  Cos/1 -> Product3/1, Product/1
  Sin/1 -> Product2/1, Product1/1
  Fy_fL/1 -> Product3/2, Product1/2
  Product/1 -> Add/1
  Product1/1 -> Add/2
  Add/1 -> Fx_fL_1/1
  Product2/1 -> Add1/1
  Product3/1 -> Add1/2
  Add1/1 -> Fy_fL_1/1

== system tadpole_dynamic_open_loop1/Vehicle Model/Normal Force Distribution/Subsystem1 ==
  delta_R : Inport
  Fx_fR : Inport  Port=2
  Fy_fR : Inport  Port=3
  Add : Sum  Inputs=+-
  Add1 : Sum
  Cos : Trigonometry  Operator=cos
  Product{,1..3} (4 alike) : Product
  Sin : Trigonometry
  Fx_fR_1 : Outport  VectorParamsAs1DForOutWhenUnconnected=off
  Fy_fR_1 : Outport  Port=2  VectorParamsAs1DForOutWhenUnconnected=off
  wires:
  delta_R/1 -> Sin/1, Cos/1
  Fx_fR/1 -> Product/2, Product2/2
  Cos/1 -> Product3/1, Product/1
  Sin/1 -> Product2/1, Product1/1
  Fy_fR/1 -> Product3/2, Product1/2
  Product/1 -> Add/1
  Product1/1 -> Add/2
  Add/1 -> Fx_fR_1/1
  Product2/1 -> Add1/1
  Product3/1 -> Add1/2
  Add1/1 -> Fy_fR_1/1

== system tadpole_dynamic_open_loop1/Vehicle Model/Speed PID controler /If Action Subsystem ==
  In1 : Inport
  Action Port : ActionPort  ActionPortLabel=if(u1 > 0)
  Out1 : Outport  VectorParamsAs1DForOutWhenUnconnected=off
  wires:
  In1/1 -> Out1/1

== system tadpole_dynamic_open_loop1/Vehicle Model/Speed PID controler /If Action Subsystem1 ==
  In1 : Inport
  Action Port : ActionPort  ActionPortLabel=else
  Out1 : Outport  VectorParamsAs1DForOutWhenUnconnected=off
  wires:
  In1/1 -> Out1/1

== system tadpole_dynamic_open_loop1/Vehicle Model/Speed PID controler /PID ==
  R(s) : Inport
  Add : Sum  Inputs=+++
  Derivative : Derivative
  Integrator : Integrator
  Kd : Gain  Gain=0
  Ki : Gain  Gain=0
  Kp : Gain  Gain=200
  C(s) : Outport  VectorParamsAs1DForOutWhenUnconnected=off
  wires:
  Derivative/1 -> Add/3
  Ki/1 -> Integrator/1
  Kp/1 -> Add/1
  R(s)/1 -> Kd/1, Ki/1, Kp/1
  Add/1 -> C(s)/1
  Kd/1 -> Derivative/1
  Integrator/1 -> Add/2

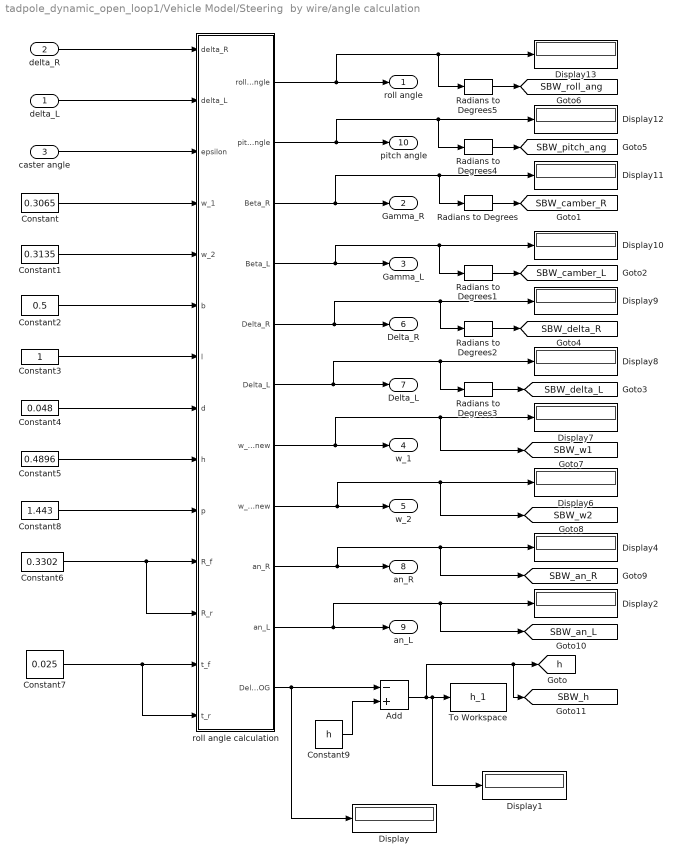
== system tadpole_dynamic_open_loop1/Vehicle Model/Steering  by wire/angle calculation ==
  delta_L : Inport
  delta_R : Inport  Port=2
  caster angle : Inport  Port=3
  Add : Sum  Inputs=-+
  Constant : Constant  Value=0.3065
  Constant1 : Constant  Value=0.3135
  Constant2 : Constant  Value=0.5
  Constant3 : Constant
  Constant4 : Constant  Value=0.048
  Constant5 : Constant  Value=0.4896
  Constant6 : Constant  Value=0.3302
  Constant7 : Constant  Value=0.025
  Constant8 : Constant  Value=1.443
  Constant9 : Constant  Value=h
  Display{,1..2,4,6..13} (12 alike) : Display
  Radians to Degrees{,1..5} (6 alike) : simulink_extras/Transformations/Radians to Degrees
  To Workspace : ToWorkspace  VariableName=h_1  SaveFormat=Timeseries  SampleTime=-1
  roll angle calculation : MATLAB Function  TreatAsAtomicUnit=on
  roll angle : Outport  VectorParamsAs1DForOutWhenUnconnected=off
  Gamma_R : Outport  Port=2  VectorParamsAs1DForOutWhenUnconnected=off
  Gamma_L : Outport  Port=3  VectorParamsAs1DForOutWhenUnconnected=off
  w_1 : Outport  Port=4  VectorParamsAs1DForOutWhenUnconnected=off
  w_2 : Outport  Port=5  VectorParamsAs1DForOutWhenUnconnected=off
  Delta_R : Outport  Port=6  VectorParamsAs1DForOutWhenUnconnected=off
  Delta_L : Outport  Port=7  VectorParamsAs1DForOutWhenUnconnected=off
  an_R : Outport  Port=8  VectorParamsAs1DForOutWhenUnconnected=off
  an_L : Outport  Port=9  VectorParamsAs1DForOutWhenUnconnected=off
  pitch angle : Outport  Port=10  VectorParamsAs1DForOutWhenUnconnected=off
  tag scope: SBW_an_L=global, SBW_an_R=global, SBW_camber_L=global, SBW_camber_R=global, SBW_delta_L=global, SBW_delta_R=global, SBW_h=global, SBW_pitch_ang=global, SBW_roll_ang=global, SBW_w1=global, SBW_w2=global, h=global
  wires:
  delta_L/1 -> roll angle calculation/2(delta_L)
  Constant5/1 -> roll angle calculation/9(h)
  roll angle calculation/3(Beta_R) -> Gamma_R/1, Radians to Degrees/1, Display11/1
  delta_R/1 -> roll angle calculation/1(delta_R)
  roll angle calculation/10(an_L) -> an_L/1, [SBW_an_L], Display2/1
  roll angle calculation/5(Delta_R) -> Radians to Degrees2/1, Display9/1, Delta_R/1
  roll angle calculation/9(an_R) -> [SBW_an_R], Display4/1, an_R/1
  roll angle calculation/7(w_1_new) -> [SBW_w1], Display7/1, w_1/1
  caster angle/1 -> roll angle calculation/3(epsilon)
  Constant/1 -> roll angle calculation/4(w_1)
  Constant3/1 -> roll angle calculation/7(l)
  Constant2/1 -> roll angle calculation/6(b)
  roll angle calculation/8(w_2_new) -> [SBW_w2], Display6/1, w_2/1
  Constant4/1 -> roll angle calculation/8(d)
  Constant6/1 -> roll angle calculation/11(R_f), roll angle calculation/12(R_r)
  Constant8/1 -> roll angle calculation/10(p)
  Constant1/1 -> roll angle calculation/5(w_2)
  roll angle calculation/1(roll_angle) -> Radians to Degrees5/1, Display13/1, roll angle/1
  Constant7/1 -> roll angle calculation/14(t_r), roll angle calculation/13(t_f)
  roll angle calculation/2(pitch_angle) -> Radians to Degrees4/1, Display12/1, pitch angle/1
  roll angle calculation/11(Delta_h_COG) -> Display/1, Add/1
  Constant9/1 -> Add/2
  Add/1 -> [SBW_h], [h], Display1/1, To Workspace/1
  Radians to Degrees/1 -> [SBW_camber_R]
  roll angle calculation/4(Beta_L) -> Radians to Degrees1/1, Display10/1, Gamma_L/1
  Radians to Degrees1/1 -> [SBW_camber_L]
  Radians to Degrees2/1 -> [SBW_delta_R]
  Radians to Degrees3/1 -> [SBW_delta_L]
  roll angle calculation/6(Delta_L) -> Radians to Degrees3/1, Display8/1, Delta_L/1
  Radians to Degrees4/1 -> [SBW_pitch_ang]
  Radians to Degrees5/1 -> [SBW_roll_ang]

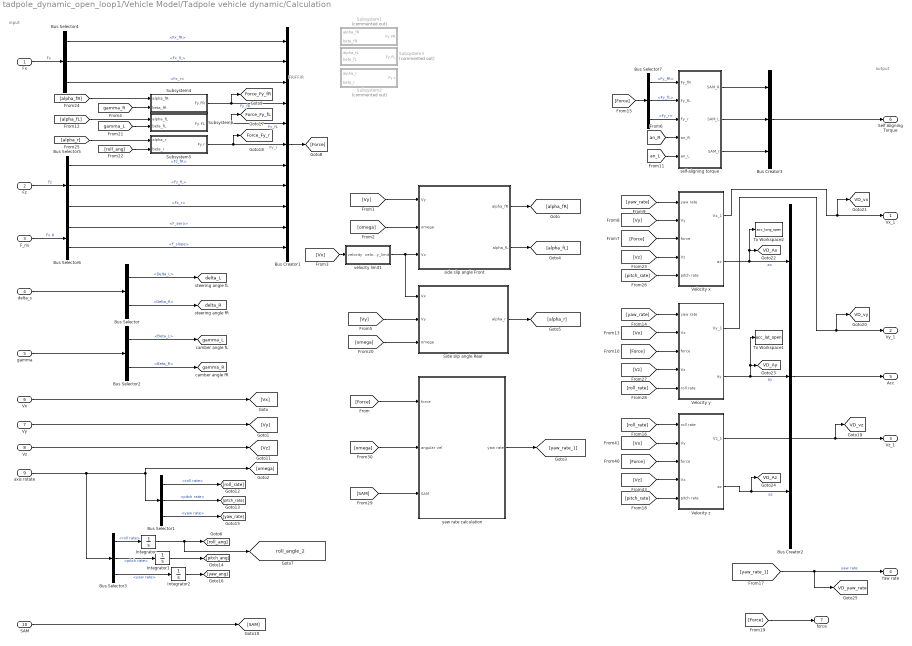
== system tadpole_dynamic_open_loop1/Vehicle Model/Tadpole vehicle dynamic/Calculation ==
  note: input
  note: output
  note: FR/FF/R
  Fx : Inport
  Fz : Inport  Port=2
  F_ris : Inport  Port=3
  delta_s : Inport  Port=4
  gamma : Inport  Port=5
  Vx : Inport  Port=6
  Vy : Inport  Port=7
  Vz : Inport  Port=8
  axis rotate : Inport  Port=9
  SAM : Inport  Port=10
  Bus Creator1 : BusCreator  Inputs=11
  Bus Creator2 : BusCreator  Inputs=3
  Bus Creator3 : BusCreator  Inputs=3
  Bus Selector : BusSelector  OutputSignals=Delta_L,Delta_R
  Bus Selector1 : BusSelector  OutputSignals=roll rate,pitch rate,yaw rate
  Bus Selector2 : BusSelector  OutputSignals=Beta_L,Beta_R
  Bus Selector3 : BusSelector  OutputSignals=roll rate,pitch rate,yaw rate
  Bus Selector4 : BusSelector  OutputSignals=Fx_fR,Fx_fL,Fx_r
  Bus Selector5 : BusSelector  OutputSignals=Fz_fR,Fz_fL,Fz_r
  Bus Selector6 : BusSelector  OutputSignals=F_aero,F_slope
  Bus Selector7 : BusSelector  OutputSignals=Fy_fR,Fy_fL,Fy_r
  Integrator : Integrator
  Integrator1 : Integrator
  Integrator2 : Integrator
  Side slip angle Rear : Subsystem
  Subsystem1 : Subsystem  Commented=on
  Subsystem2 : Subsystem  Commented=on
  Subsystem3 : Subsystem  Commented=on
  Subsystem4 : Subsystem
  Subsystem5 : Subsystem
  Subsystem6 : Subsystem
  To Workspace1 : ToWorkspace  VariableName=acc_lat_open  SaveFormat=Timeseries  SampleTime=-1
  To Workspace2 : ToWorkspace  VariableName=acc_long_open  SaveFormat=Timeseries  SampleTime=-1
  Velocity x : Subsystem
  Velocity y : Subsystem
  Velocity z : Subsystem
  self-aligning torque : Subsystem
  side slip angle Front : Subsystem
  velocity limit1 : Subsystem
  yaw rate calculation : Subsystem
  Vx_1 : Outport  VectorParamsAs1DForOutWhenUnconnected=off
  Vy_1 : Outport  Port=2  VectorParamsAs1DForOutWhenUnconnected=off
  Vz_1 : Outport  Port=3  VectorParamsAs1DForOutWhenUnconnected=off
  Yaw rate : Outport  Port=4  VectorParamsAs1DForOutWhenUnconnected=off
  Acc : Outport  Port=5  VectorParamsAs1DForOutWhenUnconnected=off
  Self Aligning Torque : Outport  Port=6  VectorParamsAs1DForOutWhenUnconnected=off
  force : Outport  Port=7  VectorParamsAs1DForOutWhenUnconnected=off
  tag scope: Force_Fy_fL=global, Force_Fy_fR=global, Force_Fy_r=global, VD_Ax=global, VD_Ay=global, VD_Az=global, VD_vx=global, VD_vy=global, VD_vz=global, VD_yaw_rate=global, delta_L=global, delta_R=global, gamma_L=global, gamma_R=global, roll_angle_2=global
  wires:
  delta_s/1 -> Bus Selector/1
  Bus Selector/1 -> [delta_L]  "<Delta_L>"
  Bus Selector/2 -> [delta_R]  "<Delta_R>"
  Vx/1 -> [Vx]
  Vy/1 -> [Vy]
  [Force] -> yaw rate calculation/1(force)
  yaw rate calculation/1(yaw rate) -> [yaw_rate_1]
  Bus Creator1/1 -> [Force]
  [Vy] -> side slip angle Front/1(Vy)
  [omega] -> side slip angle Front/2(omega)
  [omega] -> Side slip angle Rear/3(omega)
  [Vy] -> Side slip angle Rear/2(Vy)
  side slip angle Front/1(alpha_fR) -> [alpha_fR]
  side slip angle Front/2(alpha_fL) -> [alpha_fL]
  Side slip angle Rear/1(alpha_r) -> [alpha_r]
  self-aligning torque/1(SAM_R) -> Bus Creator3/1
  self-aligning torque/2(SAM_L) -> Bus Creator3/2
  [Vx] -> velocity limit1/1("velocity ")
  velocity limit1/1("velocity_limit ") -> Side slip angle Rear/1(Vx), side slip angle Front/3(Vx)
  [yaw_rate] -> Velocity x/1(yaw rate)
  [Vy] -> Velocity x/2(Vy)
  [Force] -> Velocity x/3("force ")
  Velocity x/1(Vx_1) -> [VD_vx], Vx_1/1
  Velocity x/2(ax) -> To Workspace2/1, [VD_Ax], Bus Creator2/1  "ax"
  [Force] -> Velocity y/3("force ")
  Velocity y/1(Vy_1) -> [VD_vy], Vy_1/1
  [yaw_rate] -> Velocity y/1(yaw rate)
  [Vx] -> Velocity y/2(Vx)
  [yaw_rate_1] -> [VD_yaw_rate], Yaw rate/1  "yaw rate"
  SAM/1 -> [SAM]
  [Vz] -> Velocity x/4(Vz)
  [pitch_rate] -> Velocity x/5(pitch rate)
  Vz/1 -> [Vz]
  Bus Selector1/1 -> [roll_rate]  "<roll rate>"
  Bus Selector1/2 -> [pitch_rate]  "<pitch rate>"
  Bus Selector1/3 -> [yaw_rate]  "<yaw rate>"
  [Vz] -> Velocity y/4(Vz)
  [roll_rate] -> Velocity y/5(roll rate)
  [SAM] -> yaw rate calculation/3(SAM)
  [omega] -> yaw rate calculation/2(angular vel)
  self-aligning torque/3(SAM_r) -> Bus Creator3/3
  Velocity z/1(Vz_1) -> [VD_vz], Vz_1/1
  [Vx] -> Velocity z/2(Vy)
  [pitch_rate] -> Velocity z/5(pitch rate)
  [roll_rate] -> Velocity z/1(roll rate)
  [Force] -> Velocity z/3("force ")
  Velocity z/2(az) -> [VD_Az], Bus Creator2/3  "az"
  [Vz] -> Velocity z/4(Vx)
  Bus Creator2/1 -> Acc/1
  Bus Creator3/1 -> Self Aligning Torque/1
  gamma/1 -> Bus Selector2/1
  Bus Selector2/1 -> [gamma_L]  "<Beta_L>"
  Bus Selector2/2 -> [gamma_R]  "<Beta_R>"
  Bus Selector3/3 -> Integrator2/1  "<yaw rate>"
  Bus Selector3/2 -> Integrator1/1  "<pitch rate>"
  Bus Selector3/1 -> Integrator/1  "<roll rate>"
  axis rotate/1 -> Bus Selector3/1, [omega], Bus Selector1/1
  Integrator/1 -> [roll_angle_2], [roll_ang]
  Integrator1/1 -> [pitch_ang]
  Integrator2/1 -> [yaw_ang]
  Fx/1 -> Bus Selector4/1  "Fx"
  Bus Selector4/1 -> Bus Creator1/1  "<Fx_fR>"
  Bus Selector4/2 -> Bus Creator1/2  "<Fx_fL>"
  Bus Selector4/3 -> Bus Creator1/3  "<Fx_r>"
  [gamma_L] -> Subsystem6/2(beta_fL)
  [alpha_fR] -> Subsystem4/1(alpha_fR)
  [gamma_R] -> Subsystem4/2(beta_fR)
  [alpha_fL] -> Subsystem6/1(alpha_fL)
  [roll_ang] -> Subsystem5/2(beta_r)
  [alpha_r] -> Subsystem5/1(alpha_r)
  Subsystem4/1(Fy.FR) -> [Force_Fy_fR], Bus Creator1/4  "Fy_fR"
  Subsystem6/1(Fy.FL) -> [Force_Fy_fL], Bus Creator1/5  "Fy_fL"
  Subsystem5/1(Fy.r) -> [Force_Fy_r], Bus Creator1/6  "Fy_r"
  Fz/1 -> Bus Selector5/1  "Fz"
  Bus Selector5/2 -> Bus Creator1/8  "<Fz_fL>"
  Bus Selector5/1 -> Bus Creator1/7  "<Fz_fR>"
  Bus Selector5/3 -> Bus Creator1/9  "<Fz_r>"
  F_ris/1 -> Bus Selector6/1  "Fx.R"
  Bus Selector6/1 -> Bus Creator1/10  "<F_aero>"
  Bus Selector6/2 -> Bus Creator1/11  "<F_slope>"
  [Force] -> force/1
  [an_R] -> self-aligning torque/4(an_R)
  [an_L] -> self-aligning torque/5(an_L)
  [Force] -> Bus Selector7/1
  Bus Selector7/1 -> self-aligning torque/1(Fy_fR)  "<Fy_fR>"
  Bus Selector7/2 -> self-aligning torque/2(Fy_fL)  "<Fy_fL>"
  Bus Selector7/3 -> self-aligning torque/3(Fy_r)  "<Fy_r>"
  Velocity y/2(ay) -> To Workspace1/1, [VD_Ay], Bus Creator2/2  "ay"

== system tadpole_dynamic_open_loop1/Vehicle Model/Tadpole vehicle dynamic/local to global ==
  Vy : Inport
  yaw rate : Inport  Port=2
  Vx : Inport  Port=3
  Add : Sum
  Add1 : Sum
  Gain : Gain  Gain=-1
  Integrator : Integrator
  Multiply{,1..3} (4 alike) : Product
  Sin : Trigonometry
  Sin1 : Trigonometry  Operator=cos
  absolute x dot : Outport  VectorParamsAs1DForOutWhenUnconnected=off
  absolute y dot : Outport  Port=2  VectorParamsAs1DForOutWhenUnconnected=off
  tag scope: VD_yaw_angle=global
  wires:
  Gain/1 -> Add/2
  Vx/1 -> Multiply/2, Multiply2/2
  Multiply1/1 -> Gain/1
  Sin/1 -> Multiply2/1, Multiply1/1
  Multiply3/1 -> Add1/2
  Integrator/1 -> [VD_yaw_angle], [A]
  Sin1/1 -> Multiply3/1, Multiply/1
  Multiply/1 -> Add/1
  Vy/1 -> Multiply3/2, Multiply1/2
  Add/1 -> absolute x dot/1  "absolute x dot"
  [A] -> Sin1/1, Sin/1
  Multiply2/1 -> Add1/1
  Add1/1 -> absolute y dot/1
  yaw rate/1 -> Integrator/1

== system tadpole_dynamic_open_loop1/Vehicle Model/resistance calculation/Aerodynamic Drag Force ==
  Vx : Inport
  Add : Sum
  Air density : Constant  Value=rho
  Constant : Constant  Value=V_wind
  Constant5 : Constant  Value=0.5
  Constant6 : Constant  Value=2
  "Drag coefficient " : Constant  Value=Cd
  Front Area : Constant  Value=FA
  Gain : Gain  Gain=-1
  Math Function : Math  Operator=pow  SaturateOnIntegerOverflow=on
  Product1 : Product  Inputs=6
  Sign : Signum
  F_aero : Outport  VectorParamsAs1DForOutWhenUnconnected=off
  wires:
  Add/1 -> Math Function/1, Sign/1
  Constant6/1 -> Math Function/2
  "Drag coefficient "/1 -> Product1/3
  Product1/1 -> F_aero/1
  Math Function/1 -> Product1/5
  Constant5/1 -> Product1/1
  Air density/1 -> Product1/4
  Front Area/1 -> Product1/2
  Sign/1 -> Gain/1
  Gain/1 -> Product1/6
  Vx/1 -> Add/1
  Constant/1 -> Add/2

== system tadpole_dynamic_open_loop1/Vehicle Model/resistance calculation/Rear Traction add up ==
  break : Inport
  motor : Inport  Port=2
  V sign : Inport  Port=3
  Abs : Abs
  Abs1 : Abs
  Fm<0 : Subsystem  TreatAsAtomicUnit=on
  Fm>=0 : Subsystem  TreatAsAtomicUnit=on
  If (check motor sign) : If  IfExpression=u1 >= 0
  Merge : Merge
  Rear Traction : Outport  VectorParamsAs1DForOutWhenUnconnected=off
  wires:
  Abs/1 -> Fm<0/1(|break|), Fm>=0/1(|break|)  "break"
  motor/1 -> If (check motor sign)/1, Abs1/1
  Abs1/1 -> Fm<0/2(|motor|), Fm>=0/2(|motor|)  "motor"
  break/1 -> Abs/1
  If (check motor sign)/1 -> Fm>=0/Action
  If (check motor sign)/2 -> Fm<0/Action
  Fm>=0/1(Out1) -> Merge/1
  Fm<0/1(Out1) -> Merge/2
  Merge/1 -> Rear Traction/1
  V sign/1 -> Fm<0/3("velocity sign "), Fm>=0/3("velocity sign ")  "velocity sign"
